simulink model "series_link_blance_leg"  (R2023b)
settings: Solver=ode45  StartTime=0.0  StopTime=20  MaxStep=0.2  RelTol=1e-3
values from neighbouring files (symbols this model uses):
  a11 = polyfit(leg,k11,2)    [series_get_k.m]
  a12 = polyfit(leg,k12,2)    [series_get_k.m]
  a13 = polyfit(leg,k13,1)    [series_get_k.m]
  a14 = polyfit(leg,k14,2)    [series_get_k.m]
  N = mp*diff(x + L*sin(theta),t,2)    [series_get_k1_length.m]
undefined symbols (not defined in the file or in its folder): X, Y, Z
libraries: sm_lib x59, nesl_utility x10, slpidlib x2, matrix_library x2
(part 1 of 3)
settings Model: SimulationMode=accelerator  Creator=Hhop  LastModifiedBy=陈亦杨
settings SolverCC: MinimalZcImpactIntegration=on
settings OptimizationCC: ReuseModelBlockBuffer=off
settings DebuggingCC: ReadBeforeWriteMsg=DisableAll  WriteAfterWriteMsg=DisableAll  WriteAfterReadMsg=DisableAll  MultiTaskDSMMsg=none
settings ModelReferenceCC: UpdateModelReferenceTargets=IfOutOfDate
settings SFSimCC: SFSimEcho=off

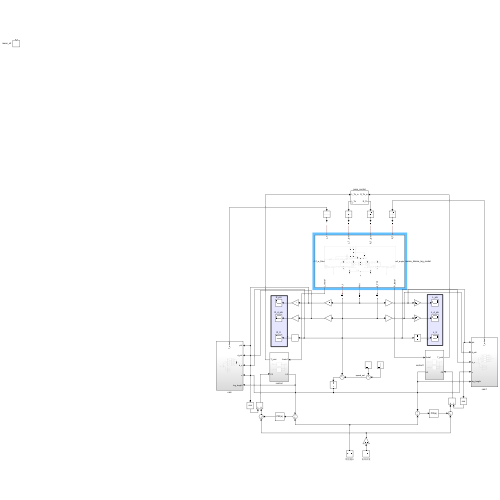
[thumbnail: Simulink's stored preview of the top-level diagram]
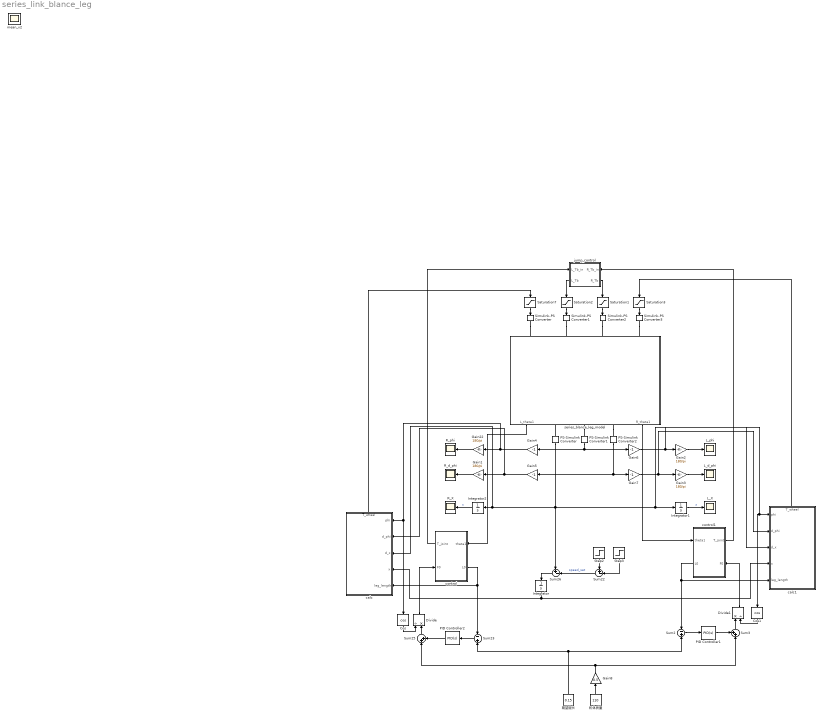
== system series_link_blance_leg ==
  Cos : Trigonometry  Operator=cos
  Cos1 : Trigonometry  Operator=cos
  Divide : Product  Inputs=/*
  Divide1 : Product  Inputs=*/
  Gain{1..3,22} (4 alike) : Gain  Gain=180/pi
  Gain{4..7} (4 alike) : Gain  Gain=-1
  Gain8 : Gain  Gain=0.5
  Integrator : Integrator
  Integrator1 : Integrator
  Integrator2 : Integrator
  L_X : Scope
  L_d_phi : Scope
  L_phi : Scope
  PID Controller1 : slpidlib/PID Controller  Controller=PID  Form=Parallel  TimeDomain=Continuous-time  UseExternalTs=off  SampleTime=-1  IntegratorMethod=Forward Euler  FilterMethod=Forward Euler  ControllerParametersSource=internal  P=200  I=0  UseKiTs=off  D=200  N=100  UseFilter=on  TunerSelectOption=Transfer Function Based (PID Tuner App)  InitialConditionSource=internal  InitialConditionForIntegrator=0  InitialConditionForFilter=0  DifferentiatorICPrevScaledInput=0  ExternalReset=none  TrackingMode=off  Kt=1  LimitOutput=off  SatLimitsSource=internal  UpperSaturationLimit=inf  LowerSaturationLimit=-inf  LinearizeAsGain=on  AntiWindupMode=none  Kb=1  LimitIntegrator=off  UpperIntegratorSaturationLimit=inf  LowerIntegratorSaturationLimit=-inf  POutMin=[]  POutMax=[]  IOutMin=[]  IOutMax=[]  DOutMin=[]  DOutMax=[]  NOutMin=[]  NOutMax=[]  SumOutMin=[]  SumOutMax=[]  SaturationOutMin=[]  SaturationOutMax=[]  PParamMin=[]  PParamMax=[]  IParamMin=[]  IParamMax=[]  DParamMin=[]  DParamMax=[]  NParamMin=[]  NParamMax=[]  KbParamMin=[]  KbParamMax=[]  KtParamMin=[]  KtParamMax=[]  KbOutMin=[]  KbOutMax=[]  KtOutMin=[]  KtOutMax=[]  IntegratorOutMin=[]  IntegratorOutMax=[]  FilterOutMin=[]  FilterOutMax=[]  SumI1OutMin=[]  SumI1OutMax=[]  SumI2OutMin=[]  SumI2OutMax=[]  SumI3OutMin=[]  SumI3OutMax=[]  SumI4OutMin=[]  SumI4OutMax=[]  SumDOutMin=[]  SumDOutMax=[]  DifferentiatorOutMin=[]  DifferentiatorOutMax=[]  FilterDiffOutCoefMin=[]  FilterDiffOutCoefMax=[]  ReciprocalOutMin=[]  ReciprocalOutMax=[]  SumDenOutMin=[]  SumDenOutMax=[]  SumNumOutMin=[]  SumNumOutMax=[]  DivideOutMin=[]  DivideOutMax=[]  UdiffTsProdOutMin=[]  UdiffTsProdOutMax=[]  NTsProdOutMin=[]  NTsProdOutMax=[]  UintegralTsProdOutMin=[]  UintegralTsProdOutMax=[]  UngainTsProdOutMin=[]  UngainTsProdOutMax=[]  ClampingZeroOutDataTypeStr=Inherit: Inherit via back propagation  ClampingZeroOutMin=[]  ClampingZeroOutMax=[]  FilterDenConstantOutDataTypeStr=Inherit: Inherit via back propagation  FilterDenConstantOutMin=[]  FilterDenConstantOutMax=[]  PCopyOutDataTypeStr=Inherit: Inherit via back propagation  PCopyOutMin=[]  PCopyOutMax=[]  NCopyOutDataTypeStr=Inherit: Inherit via back propagation  NCopyOutMin=[]  NCopyOutMax=[]  IntegratorContinuousStateAttributes=''  IntegratorStateMustResolveToSignalObject=off  IntegratorRTWStateStorageClass=Auto  FilterContinuousStateAttributes=''  FilterStateMustResolveToSignalObject=off  FilterRTWStateStorageClass=Auto  ParallelPVariant=InternalParameters  IdealPVariant=Disabled  IVariant=InternalParameters  DVariant=InternalParameters  IntegratorVariant=Continuous  SatVariant=Disabled  AWVariant=Passthrough  PCopyVariant=Disabled  TRVariant=Disabled  FdbkBlocksVariant=Forward  IdealPFdbkVariant=Disabled  SatFdbkVariant=Disabled  DerivativeFilterVariant=ContFilter  NVariant=InternalParameters  NCopyVariant=Disabled  FilterICVariant=InternalICsFilter  IntegratorICVariant=InternalICs  ExternalResetVariant=Disabled  TRSumVariant=Passthrough  SumFdbkVariant=Disabled  SumVariant=Sum_PID  TsampFilterVariant=InternalTs  TsampNgainVariant=Passthrough  TsampIntegralVariant=Disabled_SignalSpec  ExternalSaturationOutDataTypeStr=Inherit: Same as second input
  PID Controller2 : slpidlib/PID Controller  Controller=PID  Form=Parallel  TimeDomain=Continuous-time  UseExternalTs=off  SampleTime=-1  IntegratorMethod=Forward Euler  FilterMethod=Forward Euler  ControllerParametersSource=internal  P=200  I=0  UseKiTs=off  D=200  N=100  UseFilter=on  TunerSelectOption=Transfer Function Based (PID Tuner App)  InitialConditionSource=internal  InitialConditionForIntegrator=0  InitialConditionForFilter=0  DifferentiatorICPrevScaledInput=0  ExternalReset=none  TrackingMode=off  Kt=1  LimitOutput=off  SatLimitsSource=internal  UpperSaturationLimit=inf  LowerSaturationLimit=-inf  LinearizeAsGain=on  AntiWindupMode=none  Kb=1  LimitIntegrator=off  UpperIntegratorSaturationLimit=inf  LowerIntegratorSaturationLimit=-inf  POutMin=[]  POutMax=[]  IOutMin=[]  IOutMax=[]  DOutMin=[]  DOutMax=[]  NOutMin=[]  NOutMax=[]  SumOutMin=[]  SumOutMax=[]  SaturationOutMin=[]  SaturationOutMax=[]  PParamMin=[]  PParamMax=[]  IParamMin=[]  IParamMax=[]  DParamMin=[]  DParamMax=[]  NParamMin=[]  NParamMax=[]  KbParamMin=[]  KbParamMax=[]  KtParamMin=[]  KtParamMax=[]  KbOutMin=[]  KbOutMax=[]  KtOutMin=[]  KtOutMax=[]  IntegratorOutMin=[]  IntegratorOutMax=[]  FilterOutMin=[]  FilterOutMax=[]  SumI1OutMin=[]  SumI1OutMax=[]  SumI2OutMin=[]  SumI2OutMax=[]  SumI3OutMin=[]  SumI3OutMax=[]  SumI4OutMin=[]  SumI4OutMax=[]  SumDOutMin=[]  SumDOutMax=[]  DifferentiatorOutMin=[]  DifferentiatorOutMax=[]  FilterDiffOutCoefMin=[]  FilterDiffOutCoefMax=[]  ReciprocalOutMin=[]  ReciprocalOutMax=[]  SumDenOutMin=[]  SumDenOutMax=[]  SumNumOutMin=[]  SumNumOutMax=[]  DivideOutMin=[]  DivideOutMax=[]  UdiffTsProdOutMin=[]  UdiffTsProdOutMax=[]  NTsProdOutMin=[]  NTsProdOutMax=[]  UintegralTsProdOutMin=[]  UintegralTsProdOutMax=[]  UngainTsProdOutMin=[]  UngainTsProdOutMax=[]  ClampingZeroOutDataTypeStr=Inherit: Inherit via back propagation  ClampingZeroOutMin=[]  ClampingZeroOutMax=[]  FilterDenConstantOutDataTypeStr=Inherit: Inherit via back propagation  FilterDenConstantOutMin=[]  FilterDenConstantOutMax=[]  PCopyOutDataTypeStr=Inherit: Inherit via back propagation  PCopyOutMin=[]  PCopyOutMax=[]  NCopyOutDataTypeStr=Inherit: Inherit via back propagation  NCopyOutMin=[]  NCopyOutMax=[]  IntegratorContinuousStateAttributes=''  IntegratorStateMustResolveToSignalObject=off  IntegratorRTWStateStorageClass=Auto  FilterContinuousStateAttributes=''  FilterStateMustResolveToSignalObject=off  FilterRTWStateStorageClass=Auto  ParallelPVariant=InternalParameters  IdealPVariant=Disabled  IVariant=InternalParameters  DVariant=InternalParameters  IntegratorVariant=Continuous  SatVariant=Disabled  AWVariant=Passthrough  PCopyVariant=Disabled  TRVariant=Disabled  FdbkBlocksVariant=Forward  IdealPFdbkVariant=Disabled  SatFdbkVariant=Disabled  DerivativeFilterVariant=ContFilter  NVariant=InternalParameters  NCopyVariant=Disabled  FilterICVariant=InternalICsFilter  IntegratorICVariant=InternalICs  ExternalResetVariant=Disabled  TRSumVariant=Passthrough  SumFdbkVariant=Disabled  SumVariant=Sum_PID  TsampFilterVariant=InternalTs  TsampNgainVariant=Passthrough  TsampIntegralVariant=Disabled_SignalSpec  ExternalSaturationOutDataTypeStr=Inherit: Same as second input
  PS-Simulink Converter : nesl_utility/PS-Simulink Converter  PhysicalDomain=network_engine_domain  SubClassName=ps_output  LeftPortType=input  RightPortType=output  PseudoPeriodic=off  Frequencies=[]  VectorFormat=inherit  Unit=inherit  AffineConversion=off
  PS-Simulink Converter1 : nesl_utility/PS-Simulink Converter  PhysicalDomain=network_engine_domain  SubClassName=ps_output  LeftPortType=input  RightPortType=output  PseudoPeriodic=off  Frequencies=[]  VectorFormat=inherit  Unit=inherit  AffineConversion=off
  PS-Simulink Converter2 : nesl_utility/PS-Simulink Converter  PhysicalDomain=network_engine_domain  SubClassName=ps_output  LeftPortType=input  RightPortType=output  PseudoPeriodic=off  Frequencies=[]  VectorFormat=inherit  Unit=inherit  AffineConversion=off
  R_X : Scope
  R_d_phi : Scope
  R_phi : Scope
  Saturation1 : Saturate  UpperLimit=80  LowerLimit=-80
  Saturation2 : Saturate  UpperLimit=80  LowerLimit=-80
  Saturation3 : Saturate  UpperLimit=9  LowerLimit=-9
  Saturation7 : Saturate  UpperLimit=9  LowerLimit=-9
  Simulink-PS Converter{,1..3} (4 alike) : nesl_utility/Simulink-PS Converter  PhysicalDomain=network_engine_domain  SubClassName=ps_input  LeftPortType=input  RightPortType=output  PseudoPeriodic=off  Frequencies=[]  NoiseDistribution=none  NoiseParameters=[]  Unit=1  AffineConversion=off  FilteringAndDerivatives=provide  SimscapeFilterOrder=1  InputFilterTimeConstant=0.001  UdotUserProvided=0
  Step2 : Step  After=2.5  SampleTime=0
  Step3 : Step  Time=5  After=2.5  SampleTime=0
  Sum2 : Sum  Inputs=-|+
  Sum22 : Sum  Inputs=+-|
  Sum23 : Sum  Inputs=-|+
  Sum25 : Sum  Inputs=|++
  Sum26 : Sum  Inputs=+-|
  Sum3 : Sum  Inputs=++|
  calc : Subsystem
      settings: PortSchema="{\"entries\":[{\"content\":{\"sides\":[{\"content\":{\"connectorIds\":[\"In1\",\"In2\",\"In3\",\"In4\",\"In5\"]},\"type\":\"ConnectorPlacement.EquallySpacedRectSide\",\"uuid\":\"055cb80c-cd03-4a8d-aef8-6b3df8c72d3f\"},{\"content\":{\"connectorIds\":[],\"side\":\"RIGHT\"},\"type\":\"ConnectorPlacement.EquallySpacedRectSide\",\"uuid\":\"5756fad1-d70f-4a11-a5af-d2f67bfb0d7e\"},{\"content\":{\"connectorIds\":[\"Out1\"],\"side\":\"TOP\"},\"type\":\"ConnectorPlacement.EquallySpacedRectSide\",\"uuid\":\"9c70cf42-10f8-4525-9406-562484abf580\"}]},\"type\":\"ConnectorPlacement.EquallySpacedConnector\",\"uuid\":\"7084d402-0e44-4d2f-8cc2-1336d196e84d\"}],\"packageUris\":[\"http://schema.mathworks.com/mf0/Connector/R2020b\"],\"version\":\"1.0\"}"
  calc1 : Subsystem
      settings: PortSchema="{\"entries\":[{\"content\":{\"sides\":[{\"content\":{\"connectorIds\":[\"In1\",\"In2\",\"In3\",\"In4\",\"In5\"]},\"type\":\"ConnectorPlacement.EquallySpacedRectSide\",\"uuid\":\"055cb80c-cd03-4a8d-aef8-6b3df8c72d3f\"},{\"content\":{\"connectorIds\":[],\"side\":\"RIGHT\"},\"type\":\"ConnectorPlacement.EquallySpacedRectSide\",\"uuid\":\"5756fad1-d70f-4a11-a5af-d2f67bfb0d7e\"},{\"content\":{\"connectorIds\":[],\"side\":\"TOP\"},\"type\":\"ConnectorPlacement.EquallySpacedRectSide\",\"uuid\":\"9c70cf42-10f8-4525-9406-562484abf580\"},{\"content\":{\"connectorIds\":[\"Out1\"],\"side\":\"BOTTOM\"},\"type\":\"ConnectorPlacement.EquallySpacedRectSide\",\"uuid\":\"92c87742-6ac6-4602-ae8a-30b7231d5549\"}]},\"type\":\"ConnectorPlacement.EquallySpacedConnector\",\"uuid\":\"7084d402-0e44-4d2f-8cc2-1336d196e84d\"}],\"packageUris\":[\"http://schema.mathworks.com/mf0/Connector/R2020b\"],\"version\":\"1.0\"}"
  control : Subsystem
      settings: PortSchema="{\"entries\":[{\"content\":{\"sides\":[{\"content\":{\"connectorIds\":[\"In1\",\"Out2\"]},\"type\":\"ConnectorPlacement.EquallySpacedRectSide\",\"uuid\":\"52f821b9-729d-47ca-ae3d-ba1c6e84da75\"},{\"content\":{\"connectorIds\":[\"Out1\",\"In2\"],\"side\":\"RIGHT\"},\"type\":\"ConnectorPlacement.EquallySpacedRectSide\",\"uuid\":\"ec3ca8e2-1b05-45bc-ab33-c724a2b4f014\"},{\"content\":{\"connectorIds\":[],\"side\":\"TOP\"},\"type\":\"ConnectorPlacement.EquallySpacedRectSide\",\"uuid\":\"0eeea9cd-7beb-490f-b411-de67521f6335\"}]},\"type\":\"ConnectorPlacement.EquallySpacedConnector\",\"uuid\":\"61a91a11-caac-45d5-80d0-d340d78a8d6f\"}],\"packageUris\":[\"http://schema.mathworks.com/mf0/Connector/R2020b\"],\"version\":\"1.0\"}"
  control1 : Subsystem
      settings: PortSchema="{\"entries\":[{\"content\":{\"sides\":[{\"content\":{\"connectorIds\":[\"In1\",\"Out2\"]},\"type\":\"ConnectorPlacement.EquallySpacedRectSide\",\"uuid\":\"52f821b9-729d-47ca-ae3d-ba1c6e84da75\"},{\"content\":{\"connectorIds\":[\"Out1\",\"In2\"],\"side\":\"RIGHT\"},\"type\":\"ConnectorPlacement.EquallySpacedRectSide\",\"uuid\":\"ec3ca8e2-1b05-45bc-ab33-c724a2b4f014\"},{\"content\":{\"connectorIds\":[],\"side\":\"TOP\"},\"type\":\"ConnectorPlacement.EquallySpacedRectSide\",\"uuid\":\"0eeea9cd-7beb-490f-b411-de67521f6335\"}]},\"type\":\"ConnectorPlacement.EquallySpacedConnector\",\"uuid\":\"61a91a11-caac-45d5-80d0-d340d78a8d6f\"}],\"packageUris\":[\"http://schema.mathworks.com/mf0/Connector/R2020b\"],\"version\":\"1.0\"}"
  jump_control : Subsystem  mask{jump_time=3}
      mask prompts: jump_time "跳跃时间"
      settings: PortSchema="{\"entries\":[{\"content\":{\"sides\":[{\"content\":{\"connectorIds\":[\"In1\",\"Out2\"]},\"type\":\"ConnectorPlacement.EquallySpacedRectSide\",\"uuid\":\"555f1eec-a1f8-4438-898b-242296387de2\"},{\"content\":{\"connectorIds\":[\"In2\",\"Out1\"],\"side\":\"RIGHT\"},\"type\":\"ConnectorPlacement.EquallySpacedRectSide\",\"uuid\":\"4e34be98-beb2-4e32-b120-d99682746887\"},{\"content\":{\"connectorIds\":[],\"side\":\"TOP\"},\"type\":\"ConnectorPlacement.EquallySpacedRectSide\",\"uuid\":\"2dbe6b4e-143a-4ee5-b634-fdf47ce3ae58\"}]},\"type\":\"ConnectorPlacement.EquallySpacedConnector\",\"uuid\":\"fd4bce8e-8918-4201-9e0d-25b1dfe9d9e9\"}],\"packageUris\":[\"http://schema.mathworks.com/mf0/Connector/R2020b\"],\"version\":\"1.0\"}"
      mask DialogControl ParameterGroupVar Prompt: 参数
  mean_x2 : Scope
  series_blance_leg_model : Subsystem
      settings: PortSchema="{\"entries\":[{\"content\":{\"sides\":[{\"content\":{\"connectorIds\":[\"LConn1\",\"LConn2\",\"LConn3\",\"LConn4\"]},\"type\":\"ConnectorPlacement.EquallySpacedRectSide\",\"uuid\":\"ed635f35-0836-4900-93e3-56fc3520c8de\"},{\"content\":{\"connectorIds\":[\"Out1\",\"RConn1\",\"RConn2\",\"RConn3\",\"Out2\"],\"side\":\"RIGHT\"},\"type\":\"ConnectorPlacement.EquallySpacedRectSide\",\"uuid\":\"bb235ec0-defd-4ad9-96f6-8533dab3fbd9\"},{\"content\":{\"connectorIds\":[\"LConn5\"],\"side\":\"TOP\"},\"type\":\"ConnectorPlacement.EquallySpacedRectSide\",\"uuid\":\"d719db37-8b3a-4344-b330-944fde418334\"},{\"content\":{\"connectorIds\":[\"RConn4\"],\"side\":\"BOTTOM\"},\"type\":\"ConnectorPlacement.EquallySpacedRectSide\",\"uuid\":\"20f9270b-6ab1-4e89-bf00-e838d12c3c13\"}]},\"type\":\"ConnectorPlacement.EquallySpacedConnector\",\"uuid\":\"a2f25b71-0047-4a2d-a238-dad76f034ab1\"}],\"packageUris\":[\"http://schema.mathworks.com/mf0/Connector/R2020b\"],\"version\":\"1.0\"}"
  期望腿长 : Constant  Value=0.15
  机体质量 : Constant  Value=110
  wires:
  Integrator2/1 -> R_X/1  "x"
  Gain22/1 -> R_phi/1
  Gain1/1 -> R_d_phi/1
  Gain3/1 -> L_d_phi/1
  Gain2/1 -> L_phi/1
  Integrator1/1 -> L_X/1  "x"
  control/2(L0) -> Sum23/1, calc/5(leg_length)
  Sum23/1 -> PID Controller2/1
  PID Controller2/1 -> Sum25/2
  control1/2(L0) -> Sum2/1, calc1/1(leg_length)
  Sum2/1 -> PID Controller1/1
  PID Controller1/1 -> Sum3/1
  期望腿长/1 -> Sum23/2, Sum2/2
  机体质量/1 -> Gain8/1
  series_blance_leg_model/1(L_theta1) -> control/1(theta1)
  series_blance_leg_model/2(R_theta1) -> control1/1(theta1)
  PS-Simulink Converter/1 -> calc1/3(d_x), Integrator1/1, Sum26/1, calc/3(d_x), Integrator2/1
  PS-Simulink Converter1/1 -> Gain4/1, Gain6/1
  PS-Simulink Converter2/1 -> Gain7/1, Gain5/1
  Sum26/1 -> Integrator/1
  Step2/1 -> Sum22/1
  Sum22/1 -> Sum26/2  "speed_set"
  Step3/1 -> Sum22/2
  Integrator/1 -> calc/4(x), calc1/2(x)
  calc/1(T_wheel) -> Saturation7/1
  calc1/1(T_wheel) -> Saturation3/1
  Saturation2/1 -> Simulink-PS Converter1/1
  Saturation1/1 -> Simulink-PS Converter2/1
  Saturation7/1 -> Simulink-PS Converter/1
  Saturation3/1 -> Simulink-PS Converter3/1
  Gain4/1 -> Cos/1, calc/1(phi), Gain22/1
  Gain5/1 -> calc/2(d_phi), Gain1/1
  Gain6/1 -> calc1/5(phi), Cos1/1, Gain2/1
  Gain7/1 -> calc1/4(d_phi), Gain3/1
  Gain8/1 -> Sum3/2, Sum25/1
  Cos/1 -> Divide/1
  Sum25/1 -> Divide/2
  Sum3/1 -> Divide1/1
  Cos1/1 -> Divide1/2
  Divide/1 -> control/2(F0)
  Divide1/1 -> control1/2(F0)
  control/1(T_joint) -> jump_control/1(L_Tb_in)
  jump_control/2(L_Tb) -> Saturation2/1
  control1/1(T_joint) -> jump_control/2(R_Tb_in)
  jump_control/1(R_Tb) -> Saturation1/1
  connections:
  PS-Simulink Converter/LConn1 -- series_blance_leg_model/RConn1
  series_blance_leg_model/RConn2 -- PS-Simulink Converter1/LConn1
  series_blance_leg_model/RConn3 -- PS-Simulink Converter2/LConn1
  Simulink-PS Converter/RConn1 -- series_blance_leg_model/LConn1
  Simulink-PS Converter1/RConn1 -- series_blance_leg_model/LConn2
  Simulink-PS Converter2/RConn1 -- series_blance_leg_model/LConn3
  Simulink-PS Converter3/RConn1 -- series_blance_leg_model/LConn4

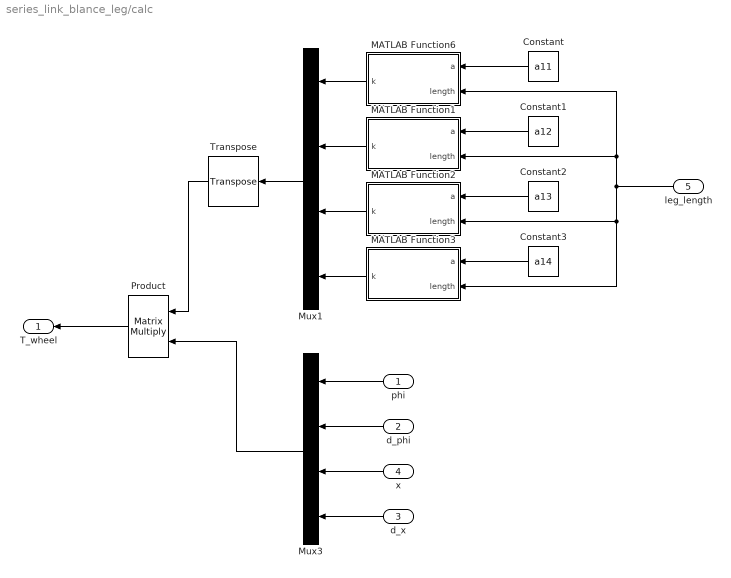
== system series_link_blance_leg/calc ==
  phi : Inport
  d_phi : Inport  Port=2
  d_x : Inport  Port=3
  x : Inport  Port=4
  leg_length : Inport  Port=5
  Constant : Constant  Value=a11
  Constant1 : Constant  Value=a12
  Constant2 : Constant  Value=a13
  Constant3 : Constant  Value=a14
  MATLAB Function1 : MATLAB Function  TreatAsAtomicUnit=on
  MATLAB Function2 : MATLAB Function  TreatAsAtomicUnit=on
  MATLAB Function3 : MATLAB Function  TreatAsAtomicUnit=on
  MATLAB Function6 : MATLAB Function  TreatAsAtomicUnit=on
  Mux1 : Mux
  Mux3 : Mux
  Product : Product  Multiplication=Matrix(*)
  Transpose : matrix_library/Transpose
  T_wheel : Outport
  wires:
  Constant/1 -> MATLAB Function6/1(a)
  Constant1/1 -> MATLAB Function1/1(a)
  Constant2/1 -> MATLAB Function2/1(a)
  Constant3/1 -> MATLAB Function3/1(a)
  leg_length/1 -> MATLAB Function6/2(length), MATLAB Function1/2(length), MATLAB Function3/2(length), MATLAB Function2/2(length)
  phi/1 -> Mux3/1
  d_phi/1 -> Mux3/2
  x/1 -> Mux3/3
  d_x/1 -> Mux3/4
  MATLAB Function6/1(k) -> Mux1/1
  MATLAB Function1/1(k) -> Mux1/2
  MATLAB Function2/1(k) -> Mux1/3
  MATLAB Function3/1(k) -> Mux1/4
  Product/1 -> T_wheel/1
  Mux3/1 -> Product/2
  Mux1/1 -> Transpose/1
  Transpose/1 -> Product/1

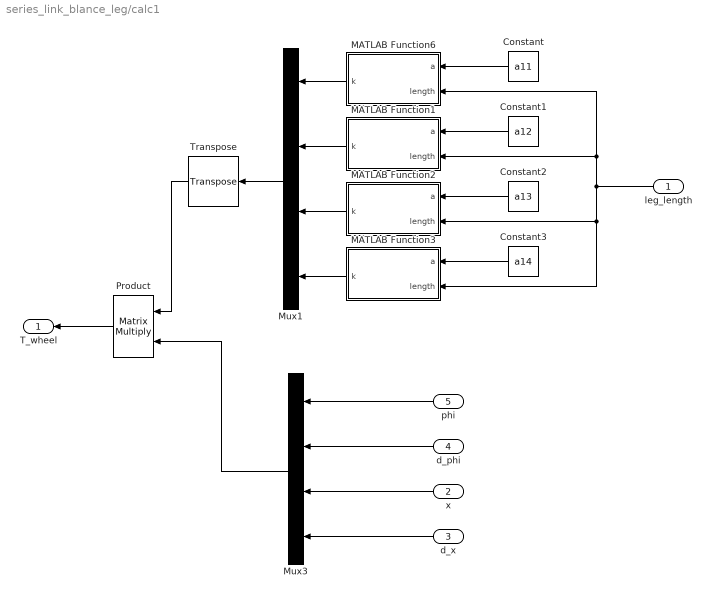
== system series_link_blance_leg/calc1 ==
  leg_length : Inport
  x : Inport  Port=2
  d_x : Inport  Port=3
  d_phi : Inport  Port=4
  phi : Inport  Port=5
  Constant : Constant  Value=a11
  Constant1 : Constant  Value=a12
  Constant2 : Constant  Value=a13
  Constant3 : Constant  Value=a14
  MATLAB Function1 : MATLAB Function  TreatAsAtomicUnit=on
  MATLAB Function2 : MATLAB Function  TreatAsAtomicUnit=on
  MATLAB Function3 : MATLAB Function  TreatAsAtomicUnit=on
  MATLAB Function6 : MATLAB Function  TreatAsAtomicUnit=on
  Mux1 : Mux
  Mux3 : Mux
  Product : Product  Multiplication=Matrix(*)
  Transpose : matrix_library/Transpose
  T_wheel : Outport
  wires:
  d_x/1 -> Mux3/4
  x/1 -> Mux3/3
  d_phi/1 -> Mux3/2
  phi/1 -> Mux3/1
  MATLAB Function1/1(k) -> Mux1/2
  Constant2/1 -> MATLAB Function2/1(a)
  MATLAB Function3/1(k) -> Mux1/4
  MATLAB Function2/1(k) -> Mux1/3
  Constant1/1 -> MATLAB Function1/1(a)
  MATLAB Function6/1(k) -> Mux1/1
  leg_length/1 -> MATLAB Function6/2(length), MATLAB Function1/2(length), MATLAB Function3/2(length), MATLAB Function2/2(length)
  Constant/1 -> MATLAB Function6/1(a)
  Constant3/1 -> MATLAB Function3/1(a)
  Mux3/1 -> Product/2
  Product/1 -> T_wheel/1
  Mux1/1 -> Transpose/1
  Transpose/1 -> Product/1

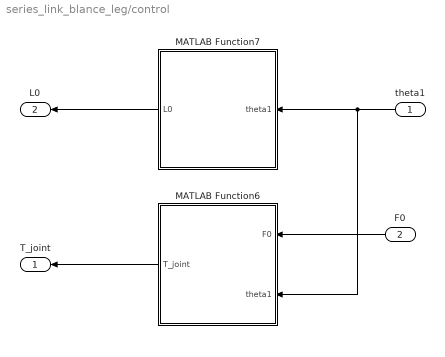
== system series_link_blance_leg/control ==
  theta1 : Inport
  F0 : Inport  Port=2
  MATLAB Function6 : MATLAB Function  TreatAsAtomicUnit=on
  MATLAB Function7 : MATLAB Function  TreatAsAtomicUnit=on
  T_joint : Outport
  L0 : Outport  Port=2
  wires:
  theta1/1 -> MATLAB Function6/2(theta1), MATLAB Function7/1(theta1)
  F0/1 -> MATLAB Function6/1(F0)
  MATLAB Function7/1(L0) -> L0/1
  MATLAB Function6/1(T_joint) -> T_joint/1

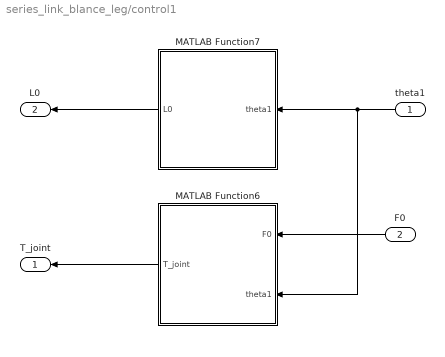
== system series_link_blance_leg/control1 ==
  theta1 : Inport
  F0 : Inport  Port=2
  MATLAB Function6 : MATLAB Function  TreatAsAtomicUnit=on
  MATLAB Function7 : MATLAB Function  TreatAsAtomicUnit=on
  T_joint : Outport
  L0 : Outport  Port=2
  wires:
  MATLAB Function6/1(T_joint) -> T_joint/1
  MATLAB Function7/1(L0) -> L0/1
  F0/1 -> MATLAB Function6/1(F0)
  theta1/1 -> MATLAB Function7/1(theta1), MATLAB Function6/2(theta1)

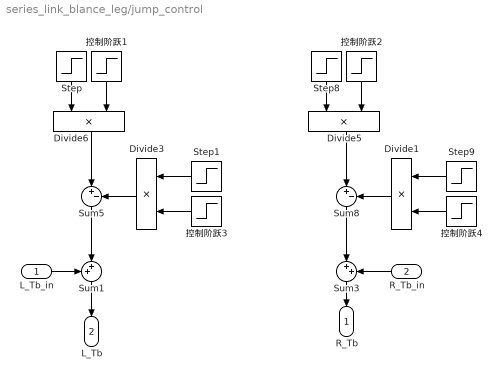
== system series_link_blance_leg/jump_control ==
  L_Tb_in : Inport
  R_Tb_in : Inport  Port=2
  Divide{1,3,5..6} (4 alike) : Product  Inputs=**
  Step : Step  Time=jump_time  After=50  SampleTime=0
  Step1 : Step  Time=jump_time+0.2  After=50  SampleTime=0
  Step8 : Step  Time=jump_time  After=50  SampleTime=0
  Step9 : Step  Time=jump_time+0.2  After=50  SampleTime=0
  Sum1 : Sum  Inputs=++|
  Sum3 : Sum  Inputs=|++
  Sum5 : Sum  Inputs=|+-
  Sum8 : Sum  Inputs=|+-
  控制阶跃1 : Step  Time=jump_time+0.15  Before=1  After=0  SampleTime=0
  控制阶跃2 : Step  Time=jump_time+0.15  Before=1  After=0  SampleTime=0
  控制阶跃3 : Step  Time=jump_time+0.4  Before=1  After=0  SampleTime=0
  控制阶跃4 : Step  Time=jump_time+0.4  Before=1  After=0  SampleTime=0
  R_Tb : Outport
  L_Tb : Outport  Port=2
  wires:
  Step9/1 -> Divide1/1
  控制阶跃4/1 -> Divide1/2
  Step1/1 -> Divide3/1
  Sum5/1 -> Sum1/2
  Step8/1 -> Divide5/1
  控制阶跃1/1 -> Divide6/2
  Divide3/1 -> Sum5/2
  Divide6/1 -> Sum5/1
  控制阶跃3/1 -> Divide3/2
  R_Tb_in/1 -> Sum3/2
  Sum8/1 -> Sum3/1
  控制阶跃2/1 -> Divide5/2
  Step/1 -> Divide6/1
  Divide5/1 -> Sum8/1
  Sum1/1 -> L_Tb/1
  L_Tb_in/1 -> Sum1/1
  Sum3/1 -> R_Tb/1
  Divide1/1 -> Sum8/2
